simulink model "dof2_test"  (Simulink 6.4)
settings: Solver=ode45  StartTime=0.0  StopTime=4  RelTol=1e-3
settings Model: Creator=Bazs  LastModifiedBy=Developer

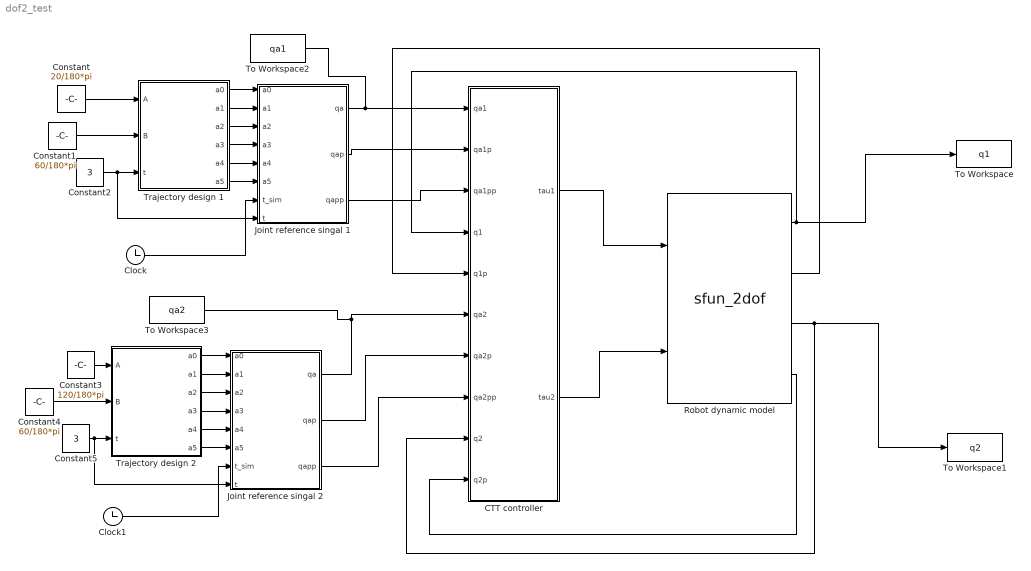
== system dof2_test ==
  CTT controller : Subsystem
  Clock : Clock
      settings: Decimation=10
  Clock1 : Clock
      settings: Decimation=10
  Constant : Constant  Value=20/180*pi  OutDataType=sfix(16)  ConRadixGroup=Use specified scaling  OutScaling=2^0  SampleTime=inf  FramePeriod=inf
  Constant1 : Constant  Value=60/180*pi  OutDataType=sfix(16)  ConRadixGroup=Use specified scaling  OutScaling=2^0  SampleTime=inf  FramePeriod=inf
  Constant2 : Constant  Value=3  OutDataType=sfix(16)  ConRadixGroup=Use specified scaling  OutScaling=2^0  SampleTime=inf  FramePeriod=inf
  Constant3 : Constant  Value=120/180*pi  OutDataType=sfix(16)  ConRadixGroup=Use specified scaling  OutScaling=2^0  SampleTime=inf  FramePeriod=inf
  Constant4 : Constant  Value=60/180*pi  OutDataType=sfix(16)  ConRadixGroup=Use specified scaling  OutScaling=2^0  SampleTime=inf  FramePeriod=inf
  Constant5 : Constant  Value=3  OutDataType=sfix(16)  ConRadixGroup=Use specified scaling  OutScaling=2^0  SampleTime=inf  FramePeriod=inf
  Joint reference singal 1 : Stateflow chart  TreatAsAtomicUnit=on
  Joint reference singal 2 : Stateflow chart  TreatAsAtomicUnit=on
  Robot dynamic model : M-S-Function  FunctionName=sfun_2dof  Parameters=10, 1, 5, 0.5, 0.2, 0.1
  To Workspace : ToWorkspace  VariableName=q1  SampleTime=-1  SaveFormat=Array
  To Workspace1 : ToWorkspace  VariableName=q2  SampleTime=-1  SaveFormat=Array
  To Workspace2 : ToWorkspace  VariableName=qa1  SampleTime=-1  SaveFormat=Array
  To Workspace3 : ToWorkspace  VariableName=qa2  SampleTime=-1  SaveFormat=Array
  Trajectory design 1 : Stateflow chart  TreatAsAtomicUnit=on
  Trajectory design 2 : Stateflow chart  TreatAsAtomicUnit=on
  wires:
  Trajectory design 1/1(a0) -> Joint reference singal 1/1(a0)
  Trajectory design 1/2(a1) -> Joint reference singal 1/2(a1)
  Trajectory design 1/3(a2) -> Joint reference singal 1/3(a2)
  Trajectory design 1/4(a3) -> Joint reference singal 1/4(a3)
  Trajectory design 1/5(a4) -> Joint reference singal 1/5(a4)
  Trajectory design 1/6(a5) -> Joint reference singal 1/6(a5)
  Constant/1 -> Trajectory design 1/1(A)
  Constant1/1 -> Trajectory design 1/2(B)
  Constant2/1 -> Trajectory design 1/3(t), Joint reference singal 1/8(t)
  Clock/1 -> Joint reference singal 1/7(t_sim)
  Trajectory design 2/1(a0) -> Joint reference singal 2/1(a0)
  Trajectory design 2/2(a1) -> Joint reference singal 2/2(a1)
  Trajectory design 2/3(a2) -> Joint reference singal 2/3(a2)
  Trajectory design 2/4(a3) -> Joint reference singal 2/4(a3)
  Trajectory design 2/5(a4) -> Joint reference singal 2/5(a4)
  Trajectory design 2/6(a5) -> Joint reference singal 2/6(a5)
  Constant3/1 -> Trajectory design 2/1(A)
  Constant4/1 -> Trajectory design 2/2(B)
  Constant5/1 -> Trajectory design 2/3(t), Joint reference singal 2/8(t)
  Clock1/1 -> Joint reference singal 2/7(t_sim)
  Joint reference singal 2/1(qa) -> CTT controller/6(qa2), To Workspace3/1
  Joint reference singal 2/2(qap) -> CTT controller/7(qa2p)
  Joint reference singal 2/3(qapp) -> CTT controller/8(qa2pp)
  CTT controller/1(tau1) -> Robot dynamic model/1
  CTT controller/2(tau2) -> Robot dynamic model/2
  Joint reference singal 1/1(qa) -> CTT controller/1(qa1), To Workspace2/1
  Joint reference singal 1/2(qap) -> CTT controller/2(qa1p)
  Joint reference singal 1/3(qapp) -> CTT controller/3(qa1pp)
  Robot dynamic model/1 -> CTT controller/4(q1), To Workspace/1
  Robot dynamic model/2 -> CTT controller/5(q1p)
  Robot dynamic model/4 -> CTT controller/10(q2p)
  Robot dynamic model/3 -> CTT controller/9(q2), To Workspace1/1

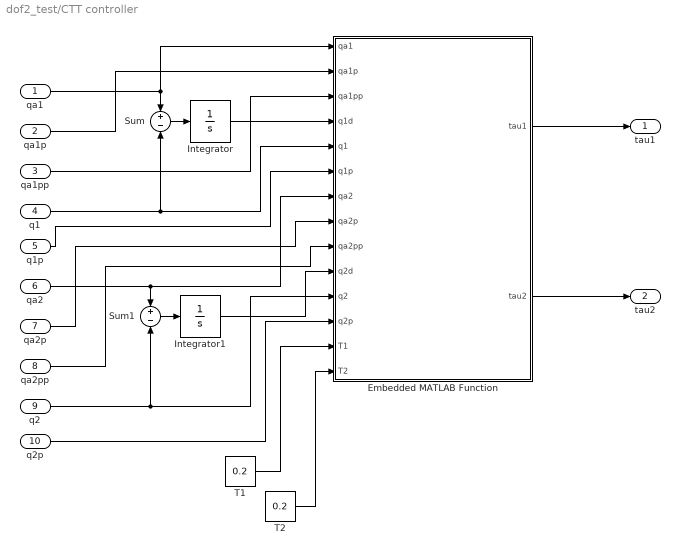
== system dof2_test/CTT controller ==
  qa1 : Inport
  qa1p : Inport  Port=2
  qa1pp : Inport  Port=3
  q1 : Inport  Port=4
  q1p : Inport  Port=5
  qa2 : Inport  Port=6
  qa2p : Inport  Port=7
  qa2pp : Inport  Port=8
  q2 : Inport  Port=9
  q2p : Inport  Port=10
  Embedded MATLAB Function : Stateflow chart  TreatAsAtomicUnit=on
  Integrator : Integrator
  Integrator1 : Integrator
  Sum : Sum  Inputs=+-
  Sum1 : Sum  Inputs=+-
  T1 : Constant  Value=0.2  OutDataType=sfix(16)  ConRadixGroup=Use specified scaling  OutScaling=2^0  SampleTime=inf  FramePeriod=inf
  T2 : Constant  Value=0.2  OutDataType=sfix(16)  ConRadixGroup=Use specified scaling  OutScaling=2^0  SampleTime=inf  FramePeriod=inf
  tau1 : Outport
  tau2 : Outport  Port=2
  wires:
  qa1/1 -> Sum/1, Embedded MATLAB Function/1(qa1)
  q1/1 -> Sum/2, Embedded MATLAB Function/5(q1)
  Sum/1 -> Integrator/1
  Integrator/1 -> Embedded MATLAB Function/4(q1d)
  qa1p/1 -> Embedded MATLAB Function/2(qa1p)
  qa1pp/1 -> Embedded MATLAB Function/3(qa1pp)
  q1p/1 -> Embedded MATLAB Function/6(q1p)
  qa2/1 -> Sum1/1, Embedded MATLAB Function/7(qa2)
  q2/1 -> Sum1/2, Embedded MATLAB Function/11(q2)
  Sum1/1 -> Integrator1/1
  Integrator1/1 -> Embedded MATLAB Function/10(q2d)
  qa2p/1 -> Embedded MATLAB Function/8(qa2p)
  qa2pp/1 -> Embedded MATLAB Function/9(qa2pp)
  q2p/1 -> Embedded MATLAB Function/12(q2p)
  T1/1 -> Embedded MATLAB Function/13(T1)
  T2/1 -> Embedded MATLAB Function/14(T2)
  Embedded MATLAB Function/1(tau1) -> tau1/1
  Embedded MATLAB Function/2(tau2) -> tau2/1

== matlab function Joint reference singal 2 ==
  data: a0 input double; a1 input double; a2 input double; a3 input double; a4 input double; a5 input double; t_sim input double; qa output double; qap output double; qapp output double; t input double
function [qa,qap,qapp] = fcn(a0,a1,a2,a3,a4,a5,t_sim,t)
% This block supports an embeddable subset of the MATLAB language.
% See the help menu for details. 
if (t_sim>t) t_sim = t;
end
T = [t_sim^5/20 t_sim^4/12 t_sim^3/6 t_sim^2/2 t_sim 1;...
    t_sim^4/4 t_sim^3/3 t_sim^2/2 t_sim 1 0;...
    t_sim^3 t_sim^2 t_sim 1 0 0];
Q = T*[a0;a1;a2;a3;a4;a5];

qa = Q(1);
qap = Q(2);
qapp = Q(3);

== matlab function CTT controller/Embedded MATLAB Function ==
  data: qa1 input double; qa1p input double; qa1pp input double; q1d input double; q1 input double; q1p input double; qa2 input double; qa2p input double; tau1 output double; qa2pp input double; q2d input double; q2 input double; q2p input double; T1 input double; tau2 output double; T2 input double
function [tau1,tau2] = fcn(qa1,qa1p,qa1pp,q1d,q1,q1p,qa2,qa2p,qa2pp,q2d,q2,q2p,T1,T2)
% This block supports an embeddable subset of the MATLAB language.
% See the help menu for details. 

l1 = 1;
l2 = 0.5;
m1 = 10;
m2 = 5;
I1 = 0.2;
I2 = 0.1;

kD1 = 3/T1;
kP1 = 3/(T1^2);
kI1 = 1/(T1^3);
kD2 = 3/T2;
kP2 = 3/(T2^2);
kI2 = 1/(T2^3);

u1 = qa1pp + kP1*(qa1-q1) + kI1*q1d + kD1*(qa1p-q1p);
u2 = qa2pp + kP2*(qa2-q2) + kI2*q2d + kD2*(qa2p-q2p);

D11 = l1^2*m1 + m2*(l1^2 + 2*l1*l2*cos(q2)+l2^2) + I1 + I2;
D12 = m2*l2*(l1*cos(q2)+l2)+I2;
D22 = m2*l2^2+I2;
D112 = -m2*l1*l2*sin(q2);
D122 = D112;

tau1 = D11*u1 + D12*u2 + 2*D112*q1p*q2p + D122*q2p^2;
tau2 = D12*u1 + D22*u2 - D112*q1p^2;

== matlab function Joint reference singal 1 ==
  data: a0 input double; a1 input double; a2 input double; a3 input double; a4 input double; a5 input double; t_sim input double; qa output double; qap output double; qapp output double; t input double
function [qa,qap,qapp] = fcn(a0,a1,a2,a3,a4,a5,t_sim,t)
% This block supports an embeddable subset of the MATLAB language.
% See the help menu for details. 
if (t_sim>t) t_sim = t;
end   
T = [t_sim^5/20 t_sim^4/12 t_sim^3/6 t_sim^2/2 t_sim 1;...
    t_sim^4/4 t_sim^3/3 t_sim^2/2 t_sim 1 0;...
    t_sim^3 t_sim^2 t_sim 1 0 0];
Q = T*[a0;a1;a2;a3;a4;a5];

qa = Q(1);
qap = Q(2);
qapp = Q(3);

== matlab function Trajectory design 1 ==
  data: A input double; B input double; t input double; a0 output double; a1 output double; a2 output double; a3 output double; a4 output double; a5 output double
function [a0,a1,a2,a3,a4,a5] = fcn(A,B,t)
% This block supports an embeddable subset of the MATLAB language.
% See the help menu for details. 
T = [t^5/20 t^4/12 t^3/6 t^2/2 t 1;t^4/4 t^3/3 t^2/2 t 1 0;t^3 t^2 t 1 0 0;0 0 0 0 0 1;0 0 0 0 1 0;0 0 0 1 0 0];
Ao = inv(T)*[B;0;0;A;0;0];
a0=Ao(1);
a1=Ao(2);
a2=Ao(3);
a3=Ao(4);
a4=Ao(5);
a5=Ao(6);

== matlab function Trajectory design 2 ==
  data: A input double; B input double; t input double; a0 output double; a1 output double; a2 output double; a3 output double; a4 output double; a5 output double
function [a0,a1,a2,a3,a4,a5] = fcn(A,B,t)
% This block supports an embeddable subset of the MATLAB language.
% See the help menu for details. 
T = [t^5/20 t^4/12 t^3/6 t^2/2 t 1;t^4/4 t^3/3 t^2/2 t 1 0;t^3 t^2 t 1 0 0;0 0 0 0 0 1;0 0 0 0 1 0;0 0 0 1 0 0];
Ao = inv(T)*[B;0;0;A;0;0];
a0=Ao(1);
a1=Ao(2);
a2=Ao(3);
a3=Ao(4);
a4=Ao(5);
a5=Ao(6);
